simulink model "Model_TranslationEngine64"  (R2022b)
settings: Solver=FixedStepDiscrete  StartTime=0.0  StopTime=5  RelTol=1e-3  EnableMultiTasking=on
InitFcn:
  | % Initialize model
  | ModelSettings=BTConfig.GetModelSettings();
  | 
  | ModelSettings.Validate();
  | 
  | ModelInit;
  | 
  | 
  | % load library data
  | GainLibrary_data;
  | % Load saved values from partition process
  | CapturedConstMask.LoadMapFromFile(bdroot)
StartFcn:
  | % make sure all the simulated RTC requests are found
  | %RTC_SIM_OBJ.ValidateREQs();
undefined symbols (not defined in the file or in its folder): AA, BPLP, Column, NumHFRefBPF, NumHFRefLPF, NumMusicChannels, Row, VolumeMuteConfig
libraries: TuneVar x925, TOP x490, FeaturePath x111, CapturedConstLib x52
(part 25 of 34)

== system Model_TranslationEngine64/ModelPreAmp/DecRate/AudioPilot35/Audiopilot_3_5/NoiseEstimationVariant/RegularNoiseEstimation/LFNoiseEstimatorCoh/SpeedBoundsAndNoiseSlew/LfNoiseSlew ==
  Attack : Subsystem
  Decay : Subsystem
  FeaturePath : FeaturePath/FeaturePath  FeatureName=Slew  IsGroup=off  GroupNumber=-1  IsModule=off  TriggerInit=[-225 44 -110 151]
      settings: SourceProductName=Bose Talaria
  SlowSlew : Subsystem
  Threshold : Subsystem  mask(Talaria Trivial Tune TOP){TriggerInit=[-265 255 -95 285], TopName=ThresholdDb, TuneName=ThresholdDb, DataTypeOut=single, MaskValue=Config.SlewThresholdDb, TunabilityNumber=1, MinValue=[], MaxValue=[], BankNumber=0, PreOverlay=false, PostOverlay=false, UseSameName=on}
      mask prompts: TriggerInit "Hidden: MoveFcn redraw"; TopName "Name:"; TuneName "Name of TuneVar:"; DataTypeOut "Data type:"; MaskValue "Default Value:"; TunabilityNumber "Tunability:"; MinValue "Min Value:"; MaxValue "Max Value:"; BankNumber "Target memory bank number:"; PreOverlay "Requires pre-overlay action:"; PostOverlay "Requires post-overlay action:"; UseSameName "Use same name for tune variable and TOP"
      mask help: The TuneTOP block encapsultes a Target Overlay Parameter, a Tune Variable, and a Trivial Translation between them.
      mask init:
      | [ok,activeTopPath,activeTunePath] = TuneTOP_Mask.Init(gcbh);
      settings: MoveFcn=TuneTOP_Mask.CB_TriggerInit(gcbh);
      mask Callback TriggerInit: TuneTOP_Mask.CB_TriggerInit(gcbh);
      mask TypeOptions TopName: TOP/TopName
      mask TypeOptions TuneName: Tune Variable/TuneName
      mask TypeOptions DataTypeOut: TOP/DataTypeOut
      mask TypeOptions MaskValue: Tune Variable/MaskValue
      mask TypeOptions TunabilityNumber: Tune Variable/TunabilityNumber
      mask Callback TunabilityNumber: TuneVarMask.CB_TunabilityNumber(gcbh);
      mask TypeOptions MinValue: Tune Variable/MinValue
      mask TypeOptions MaxValue: Tune Variable/MaxValue
      mask TypeOptions BankNumber: TOP/BankNumber
      mask TypeOptions PreOverlay: TOP/PreOverlay
      mask TypeOptions PostOverlay: TOP/PostOverlay
      mask Callback UseSameName: TuneTOP_Mask.CB_UseSameName(gcbh);
      mask DialogControl toolPanel Prompt: Tuning Tool Hints
      mask DialogControl DescriptionGroup Prompt: Description
      mask DialogControl EditDescription Prompt: Edit Description
      mask DialogControl EditDescription Callback: TuneTOP_Mask.CB_EditDescription(gcbh);
      mask DialogControl TunabilityText Prompt: Easy: Changes nearly every tuning.
      mask DialogControl AdvancedPanel Prompt: Advanced
      mask DialogControl ConvertToFullTranslation Prompt: Irreversible conversion to full translation
      mask DialogControl ConvertToFullTranslation Callback: TuneTOP_Mask.CB_ConvertToFullTranslation(gcbh);
      mask DialogControl ErrorContainer Prompt: Error Messages
      mask DialogControl ErrorText Prompt: No overlay group found. Declare one in a FeaturePath.
      mask Display:
      | % retrieve icon definition
      | [path,w,h] = TuneTOP_Mask.Icon();
      | 
      | % retrieve the block's pixel size
      | pos = get(gcbh,'position');
      | bw = pos(3) - pos(1);
      | bh = pos(4) - pos(2);
      | 
      | % draw centered icon
      | xAdj = bw/2 - w/2 + 5;
      | yAdj = bh/2 - h/2 + 4;
      | for i=1:length(path)
      | 	patch(path(i).x+xAdj, path(i).y+yAdj, path(i).rgb);
      | end
      | 
      | % show the top name or an X
      | if (exist('ok','var') && ok)
      | 	text(bw*0.5, bh*0.2, activeTopPath, 'horizontalAlignment', 'center');
      | 	patch(0,0,[1 1 1]);
      | 	patch(bw,bh,[1 1 1]);
      | else
      | 	tx=bw*0.03;
      | 	ty=bh*0.03;
      | 	patch([0 tx bw bw-tx], [ty 0 bh-ty bh], [1 0 0]);
      | 	patch([0 bw-tx bw tx], [bh-ty 0 ty bh], [1 0 0]);
      | end

== system Model_TranslationEngine64/ModelPreAmp/DecRate/AudioPilot35/Audiopilot_3_5/NoiseEstimationVariant/RegularNoiseEstimation/LFNoiseEstimatorCoh/SpeedBoundsAndNoiseSlew/SpeedBounds ==
  FeaturePath : FeaturePath/FeaturePath  FeatureName=SpeedBounds  IsGroup=off  GroupNumber=-1  IsModule=off  TriggerInit=[115 194 230 301]
      settings: SourceProductName=Bose Talaria
  axis : Subsystem  mask(Talaria Trivial Tune TOP){TriggerInit=[85 375 255 405], TopName=Axis, TuneName=Axis, DataTypeOut=single, MaskValue=Config.SpeedBoundsAxis, TunabilityNumber=1, MinValue=[], MaxValue=[], BankNumber=0, PreOverlay=false, PostOverlay=false, UseSameName=on}
      mask prompts: TriggerInit "Hidden: MoveFcn redraw"; TopName "Name:"; TuneName "Name of TuneVar:"; DataTypeOut "Data type:"; MaskValue "Default Value:"; TunabilityNumber "Tunability:"; MinValue "Min Value:"; MaxValue "Max Value:"; BankNumber "Target memory bank number:"; PreOverlay "Requires pre-overlay action:"; PostOverlay "Requires post-overlay action:"; UseSameName "Use same name for tune variable and TOP"
      mask help: The TuneTOP block encapsultes a Target Overlay Parameter, a Tune Variable, and a Trivial Translation between them.
      mask init:
      | [ok,activeTopPath,activeTunePath] = TuneTOP_Mask.Init(gcbh);
      settings: MoveFcn=TuneTOP_Mask.CB_TriggerInit(gcbh);
      mask Callback TriggerInit: TuneTOP_Mask.CB_TriggerInit(gcbh);
      mask TypeOptions TopName: TOP/TopName
      mask TypeOptions TuneName: Tune Variable/TuneName
      mask TypeOptions DataTypeOut: TOP/DataTypeOut
      mask TypeOptions MaskValue: Tune Variable/MaskValue
      mask TypeOptions TunabilityNumber: Tune Variable/TunabilityNumber
      mask Callback TunabilityNumber: TuneVarMask.CB_TunabilityNumber(gcbh);
      mask TypeOptions MinValue: Tune Variable/MinValue
      mask TypeOptions MaxValue: Tune Variable/MaxValue
      mask TypeOptions BankNumber: TOP/BankNumber
      mask TypeOptions PreOverlay: TOP/PreOverlay
      mask TypeOptions PostOverlay: TOP/PostOverlay
      mask Callback UseSameName: TuneTOP_Mask.CB_UseSameName(gcbh);
      mask DialogControl toolPanel Prompt: Tuning Tool Hints
      mask DialogControl DescriptionGroup Prompt: Description
      mask DialogControl EditDescription Prompt: Edit Description
      mask DialogControl EditDescription Callback: TuneTOP_Mask.CB_EditDescription(gcbh);
      mask DialogControl TunabilityText Prompt: Easy: Changes nearly every tuning.
      mask DialogControl AdvancedPanel Prompt: Advanced
      mask DialogControl ConvertToFullTranslation Prompt: Irreversible conversion to full translation
      mask DialogControl ConvertToFullTranslation Callback: TuneTOP_Mask.CB_ConvertToFullTranslation(gcbh);
      mask DialogControl ErrorContainer Prompt: Error Messages
      mask DialogControl ErrorText Prompt: No overlay group found. Declare one in a FeaturePath.
      mask Display:
      | % retrieve icon definition
      | [path,w,h] = TuneTOP_Mask.Icon();
      | 
      | % retrieve the block's pixel size
      | pos = get(gcbh,'position');
      | bw = pos(3) - pos(1);
      | bh = pos(4) - pos(2);
      | 
      | % draw centered icon
      | xAdj = bw/2 - w/2 + 5;
      | yAdj = bh/2 - h/2 + 4;
      | for i=1:length(path)
      | 	patch(path(i).x+xAdj, path(i).y+yAdj, path(i).rgb);
      | end
      | 
      | % show the top name or an X
      | if (exist('ok','var') && ok)
      | 	text(bw*0.5, bh*0.2, activeTopPath, 'horizontalAlignment', 'center');
      | 	patch(0,0,[1 1 1]);
      | 	patch(bw,bh,[1 1 1]);
      | else
      | 	tx=bw*0.03;
      | 	ty=bh*0.03;
      | 	patch([0 tx bw bw-tx], [ty 0 bh-ty bh], [1 0 0]);
      | 	patch([0 bw-tx bw tx], [bh-ty 0 ty bh], [1 0 0]);
      | end
  max : Subsystem  mask(Talaria Trivial Tune TOP){TriggerInit=[85 485 255 515], TopName=MaxDbspl, TuneName=MaxDbspl, DataTypeOut=single, MaskValue=Config.SpeedBoundsMaxdBSPL, TunabilityNumber=1, MinValue=[], MaxValue=[], BankNumber=0, PreOverlay=false, PostOverlay=false, UseSameName=on}
      mask prompts: TriggerInit "Hidden: MoveFcn redraw"; TopName "Name:"; TuneName "Name of TuneVar:"; DataTypeOut "Data type:"; MaskValue "Default Value:"; TunabilityNumber "Tunability:"; MinValue "Min Value:"; MaxValue "Max Value:"; BankNumber "Target memory bank number:"; PreOverlay "Requires pre-overlay action:"; PostOverlay "Requires post-overlay action:"; UseSameName "Use same name for tune variable and TOP"
      mask help: The TuneTOP block encapsultes a Target Overlay Parameter, a Tune Variable, and a Trivial Translation between them.
      mask init:
      | [ok,activeTopPath,activeTunePath] = TuneTOP_Mask.Init(gcbh);
      settings: MoveFcn=TuneTOP_Mask.CB_TriggerInit(gcbh);
      mask Callback TriggerInit: TuneTOP_Mask.CB_TriggerInit(gcbh);
      mask TypeOptions TopName: TOP/TopName
      mask TypeOptions TuneName: Tune Variable/TuneName
      mask TypeOptions DataTypeOut: TOP/DataTypeOut
      mask TypeOptions MaskValue: Tune Variable/MaskValue
      mask TypeOptions TunabilityNumber: Tune Variable/TunabilityNumber
      mask Callback TunabilityNumber: TuneVarMask.CB_TunabilityNumber(gcbh);
      mask TypeOptions MinValue: Tune Variable/MinValue
      mask TypeOptions MaxValue: Tune Variable/MaxValue
      mask TypeOptions BankNumber: TOP/BankNumber
      mask TypeOptions PreOverlay: TOP/PreOverlay
      mask TypeOptions PostOverlay: TOP/PostOverlay
      mask Callback UseSameName: TuneTOP_Mask.CB_UseSameName(gcbh);
      mask DialogControl toolPanel Prompt: Tuning Tool Hints
      mask DialogControl DescriptionGroup Prompt: Description
      mask DialogControl EditDescription Prompt: Edit Description
      mask DialogControl EditDescription Callback: TuneTOP_Mask.CB_EditDescription(gcbh);
      mask DialogControl TunabilityText Prompt: Easy: Changes nearly every tuning.
      mask DialogControl AdvancedPanel Prompt: Advanced
      mask DialogControl ConvertToFullTranslation Prompt: Irreversible conversion to full translation
      mask DialogControl ConvertToFullTranslation Callback: TuneTOP_Mask.CB_ConvertToFullTranslation(gcbh);
      mask DialogControl ErrorContainer Prompt: Error Messages
      mask DialogControl ErrorText Prompt: No overlay group found. Declare one in a FeaturePath.
      mask Display:
      | % retrieve icon definition
      | [path,w,h] = TuneTOP_Mask.Icon();
      | 
      | % retrieve the block's pixel size
      | pos = get(gcbh,'position');
      | bw = pos(3) - pos(1);
      | bh = pos(4) - pos(2);
      | 
      | % draw centered icon
      | xAdj = bw/2 - w/2 + 5;
      | yAdj = bh/2 - h/2 + 4;
      | for i=1:length(path)
      | 	patch(path(i).x+xAdj, path(i).y+yAdj, path(i).rgb);
      | end
      | 
      | % show the top name or an X
      | if (exist('ok','var') && ok)
      | 	text(bw*0.5, bh*0.2, activeTopPath, 'horizontalAlignment', 'center');
      | 	patch(0,0,[1 1 1]);
      | 	patch(bw,bh,[1 1 1]);
      | else
      | 	tx=bw*0.03;
      | 	ty=bh*0.03;
      | 	patch([0 tx bw bw-tx], [ty 0 bh-ty bh], [1 0 0]);
      | 	patch([0 bw-tx bw tx], [bh-ty 0 ty bh], [1 0 0]);
      | end
  min : Subsystem
  on : Subsystem  mask(Talaria Trivial Tune TOP){TriggerInit=[85 540 255 570], TopName=On, TuneName=On, DataTypeOut=single, MaskValue=Config.SpeedBoundsOn, TunabilityNumber=1, MinValue=[], MaxValue=[], BankNumber=0, PreOverlay=false, PostOverlay=false, UseSameName=on}
      mask prompts: TriggerInit "Hidden: MoveFcn redraw"; TopName "Name:"; TuneName "Name of TuneVar:"; DataTypeOut "Data type:"; MaskValue "Default Value:"; TunabilityNumber "Tunability:"; MinValue "Min Value:"; MaxValue "Max Value:"; BankNumber "Target memory bank number:"; PreOverlay "Requires pre-overlay action:"; PostOverlay "Requires post-overlay action:"; UseSameName "Use same name for tune variable and TOP"
      mask help: The TuneTOP block encapsultes a Target Overlay Parameter, a Tune Variable, and a Trivial Translation between them.
      mask init:
      | [ok,activeTopPath,activeTunePath] = TuneTOP_Mask.Init(gcbh);
      settings: MoveFcn=TuneTOP_Mask.CB_TriggerInit(gcbh);
      mask Callback TriggerInit: TuneTOP_Mask.CB_TriggerInit(gcbh);
      mask TypeOptions TopName: TOP/TopName
      mask TypeOptions TuneName: Tune Variable/TuneName
      mask TypeOptions DataTypeOut: TOP/DataTypeOut
      mask TypeOptions MaskValue: Tune Variable/MaskValue
      mask TypeOptions TunabilityNumber: Tune Variable/TunabilityNumber
      mask Callback TunabilityNumber: TuneVarMask.CB_TunabilityNumber(gcbh);
      mask TypeOptions MinValue: Tune Variable/MinValue
      mask TypeOptions MaxValue: Tune Variable/MaxValue
      mask TypeOptions BankNumber: TOP/BankNumber
      mask TypeOptions PreOverlay: TOP/PreOverlay
      mask TypeOptions PostOverlay: TOP/PostOverlay
      mask Callback UseSameName: TuneTOP_Mask.CB_UseSameName(gcbh);
      mask DialogControl toolPanel Prompt: Tuning Tool Hints
      mask DialogControl DescriptionGroup Prompt: Description
      mask DialogControl EditDescription Prompt: Edit Description
      mask DialogControl EditDescription Callback: TuneTOP_Mask.CB_EditDescription(gcbh);
      mask DialogControl TunabilityText Prompt: Easy: Changes nearly every tuning.
      mask DialogControl AdvancedPanel Prompt: Advanced
      mask DialogControl ConvertToFullTranslation Prompt: Irreversible conversion to full translation
      mask DialogControl ConvertToFullTranslation Callback: TuneTOP_Mask.CB_ConvertToFullTranslation(gcbh);
      mask DialogControl ErrorContainer Prompt: Error Messages
      mask DialogControl ErrorText Prompt: No overlay group found. Declare one in a FeaturePath.
      mask Display:
      | % retrieve icon definition
      | [path,w,h] = TuneTOP_Mask.Icon();
      | 
      | % retrieve the block's pixel size
      | pos = get(gcbh,'position');
      | bw = pos(3) - pos(1);
      | bh = pos(4) - pos(2);
      | 
      | % draw centered icon
      | xAdj = bw/2 - w/2 + 5;
      | yAdj = bh/2 - h/2 + 4;
      | for i=1:length(path)
      | 	patch(path(i).x+xAdj, path(i).y+yAdj, path(i).rgb);
      | end
      | 
      | % show the top name or an X
      | if (exist('ok','var') && ok)
      | 	text(bw*0.5, bh*0.2, activeTopPath, 'horizontalAlignment', 'center');
      | 	patch(0,0,[1 1 1]);
      | 	patch(bw,bh,[1 1 1]);
      | else
      | 	tx=bw*0.03;
      | 	ty=bh*0.03;
      | 	patch([0 tx bw bw-tx], [ty 0 bh-ty bh], [1 0 0]);
      | 	patch([0 bw-tx bw tx], [bh-ty 0 ty bh], [1 0 0]);
      | end

== system Model_TranslationEngine64/ModelPreAmp/DecRate/AudioPilot35/Audiopilot_3_5/NoiseEstimationVariant/RegularNoiseEstimation/RatioCalculation/APLFUP/FlagHoldTime ==
  TOP : TOP/TOP  TriggerInit=[435 27 630 73]  TopName=FlagHoldTimeSamples  DataTypeOut=single  BankNumber=0  PreOverlay=false  PostOverlay=false  Role=Automatic
      settings: SourceProductName=Bose Talaria
  TranslateTrigger : TuneVar/TranslateTrigger  TriggerInit=[306 -100 344 -45]
      settings: SourceProductName=Bose Talaria
  Tune Variable : TuneVar/TuneVar  TuneName=FlagHoldTimeS  SpecifyMaxSize=off  VariableDim=1 (Row)  MaxSize=[1 1]  TunabilityNumber=1  MinValue=[]  MaxValue=[]  TriggerInit=[-35 27 160 73]  MaskValue=Config.UpdateFlagHoldTimeSec
      settings: SourceProductName=Bose Talaria
  sec2samples : MATLAB Function  TreatAsAtomicUnit=on
  wires:
  Tune Variable/1 -> sec2samples/1(time)  "FlagHoldTimeS"
  sec2samples/1(samples) -> TOP/1
  TranslateTrigger/1 -> sec2samples/Trigger

== system Model_TranslationEngine64/ModelPreAmp/DecRate/AudioPilot35/Audiopilot_3_5/NoiseEstimationVariant/RegularNoiseEstimation/RatioCalculation/APLFUP/HfNoiseThresh ==
  TOP : TOP/TOP  TriggerInit=[440 20 585 80]  TopName=HfNoiseThreshDbspl  DataTypeOut=single  BankNumber=BankNumber  PreOverlay=PreOverlay  PostOverlay=PostOverlay  Role=Automatic
      settings: SourceProductName=Bose Talaria
  TrivialTranslation : TuneVar/TrivialTranslation  TriggerInit=[300 28 350 72]
      settings: SourceProductName=Bose Talaria
  Tune Variable : TuneVar/TuneVar  TuneName=HfNoiseThreshDbspl  SpecifyMaxSize=off  VariableDim=1 (Row)  MaxSize=[1 1]  TunabilityNumber=1  MinValue=MinValue  MaxValue=MaxValue  TriggerInit=[20 25 190 75]  MaskValue=MaskValue
      settings: SourceProductName=Bose Talaria
  wires:
  TrivialTranslation/1 -> TOP/1
  Tune Variable/1 -> TrivialTranslation/1  "HfNoiseThreshDbspl"

== system Model_TranslationEngine64/ModelPreAmp/DecRate/AudioPilot35/Audiopilot_3_5/NoiseEstimationVariant/RegularNoiseEstimation/RatioCalculation/APLFUP/LfNoiseThresh ==
  TOP : TOP/TOP  TriggerInit=[440 20 585 80]  TopName=LfNoiseThreshDbspl  DataTypeOut=single  BankNumber=BankNumber  PreOverlay=PreOverlay  PostOverlay=PostOverlay  Role=Automatic
      settings: SourceProductName=Bose Talaria
  TrivialTranslation : TuneVar/TrivialTranslation  TriggerInit=[300 28 350 72]
      settings: SourceProductName=Bose Talaria
  Tune Variable : TuneVar/TuneVar  TuneName=LfNoiseThreshDbspl  SpecifyMaxSize=off  VariableDim=1 (Row)  MaxSize=[1 1]  TunabilityNumber=1  MinValue=MinValue  MaxValue=MaxValue  TriggerInit=[20 25 190 75]  MaskValue=MaskValue
      settings: SourceProductName=Bose Talaria
  wires:
  TrivialTranslation/1 -> TOP/1
  Tune Variable/1 -> TrivialTranslation/1  "LfNoiseThreshDbspl"

== system Model_TranslationEngine64/ModelPreAmp/DecRate/AudioPilot35/Audiopilot_3_5/NoiseEstimationVariant/RegularNoiseEstimation/RatioCalculation/APLFUP/LfNoiseUpdatePeriod ==
  TOP : TOP/TOP  TriggerInit=[440 20 685 80]  TopName=LfNoiseUpdatePeriodSamples  DataTypeOut=single  BankNumber=0  PreOverlay=false  PostOverlay=false  Role=Automatic
      settings: SourceProductName=Bose Talaria
  TranslateTrigger : TuneVar/TranslateTrigger  TriggerInit=[306 -100 344 -45]
      settings: SourceProductName=Bose Talaria
  Tune Variable : TuneVar/TuneVar  TuneName=LfNoiseUpdatePeriodS  SpecifyMaxSize=off  VariableDim=1 (Row)  MaxSize=[1 1]  TunabilityNumber=1  MinValue=[]  MaxValue=[]  TriggerInit=[-100 20 145 80]  MaskValue=Config.UpdateLfNoiseUpdatePeriodSec
      settings: SourceProductName=Bose Talaria
  sec2samples : MATLAB Function  TreatAsAtomicUnit=on
  wires:
  Tune Variable/1 -> sec2samples/1(time)  "LfNoiseUpdatePeriodS"
  sec2samples/1(samples) -> TOP/1
  TranslateTrigger/1 -> sec2samples/Trigger

== system Model_TranslationEngine64/ModelPreAmp/DecRate/AudioPilot35/Audiopilot_3_5/NoiseEstimationVariant/RegularNoiseEstimation/RatioCalculation/APLFUP/LfNoiseUpdateThresh ==
  TOP : TOP/TOP  TriggerInit=[440 20 585 80]  TopName=LfNoiseUpdateThreshDb  DataTypeOut=single  BankNumber=BankNumber  PreOverlay=PreOverlay  PostOverlay=PostOverlay  Role=Automatic
      settings: SourceProductName=Bose Talaria
  TrivialTranslation : TuneVar/TrivialTranslation  TriggerInit=[300 28 350 72]
      settings: SourceProductName=Bose Talaria
  Tune Variable : TuneVar/TuneVar  TuneName=LfNoiseUpdateThreshDb  SpecifyMaxSize=off  VariableDim=1 (Row)  MaxSize=[1 1]  TunabilityNumber=1  MinValue=MinValue  MaxValue=MaxValue  TriggerInit=[20 25 190 75]  MaskValue=MaskValue
      settings: SourceProductName=Bose Talaria
  wires:
  TrivialTranslation/1 -> TOP/1
  Tune Variable/1 -> TrivialTranslation/1  "LfNoiseUpdateThreshDb"

== system Model_TranslationEngine64/ModelPreAmp/DecRate/AudioPilot35/Audiopilot_3_5/NoiseEstimationVariant/RegularNoiseEstimation/RatioCalculation/APLFUP/SpeedUpdateThresh ==
  TOP : TOP/TOP  TriggerInit=[440 20 585 80]  TopName=SpeedUpdateThreshMph  DataTypeOut=single  BankNumber=BankNumber  PreOverlay=PreOverlay  PostOverlay=PostOverlay  Role=Automatic
      settings: SourceProductName=Bose Talaria
  TrivialTranslation : TuneVar/TrivialTranslation  TriggerInit=[300 28 350 72]
      settings: SourceProductName=Bose Talaria
  Tune Variable : TuneVar/TuneVar  TuneName=SpeedUpdateThreshMph  SpecifyMaxSize=off  VariableDim=1 (Row)  MaxSize=[1 1]  TunabilityNumber=1  MinValue=MinValue  MaxValue=MaxValue  TriggerInit=[20 25 190 75]  MaskValue=MaskValue
      settings: SourceProductName=Bose Talaria
  wires:
  TrivialTranslation/1 -> TOP/1
  Tune Variable/1 -> TrivialTranslation/1  "SpeedUpdateThreshMph"

== system Model_TranslationEngine64/ModelPreAmp/DecRate/AudioPilot35/Audiopilot_3_5/NoiseEstimationVariant/RegularNoiseEstimation/RatioCalculation/RatioSlew/attack ==
  TOP : TOP/TOP  TriggerInit=[-10 87 195 133]  TopName=AttackDbPerSample  DataTypeOut=single  BankNumber=0  PreOverlay=false  PostOverlay=false  Role=Automatic
      settings: SourceProductName=Bose Talaria
  TranslateTrigger : TuneVar/TranslateTrigger  TriggerInit=[-119 -30 -81 25]
      settings: SourceProductName=Bose Talaria
  Tune Variable : TuneVar/TuneVar  TuneName=AttackDbPerS  SpecifyMaxSize=off  VariableDim=1 (Row)  MaxSize=[1 1]  TunabilityNumber=1  MinValue=[]  MaxValue=[]  TriggerInit=[-475 85 -305 135]  MaskValue=Config.SlewAttackDbpersec
      settings: SourceProductName=Bose Talaria
  sec2sample : MATLAB Function  TreatAsAtomicUnit=on
  wires:
  sec2sample/1(y) -> TOP/1
  Tune Variable/1 -> sec2sample/1(u)  "AttackDbPerS"
  TranslateTrigger/1 -> sec2sample/Trigger

== system Model_TranslationEngine64/ModelPreAmp/DecRate/AudioPilot35/Audiopilot_3_5/NoiseEstimationVariant/RegularNoiseEstimation/RatioCalculation/RatioSlew/decay ==
  TOP : TOP/TOP  TriggerInit=[-15 85 195 135]  TopName=DecayDbPerSample  DataTypeOut=single  BankNumber=0  PreOverlay=false  PostOverlay=false  Role=Automatic
      settings: SourceProductName=Bose Talaria
  TranslateTrigger : TuneVar/TranslateTrigger  TriggerInit=[-119 -30 -81 25]
      settings: SourceProductName=Bose Talaria
  Tune Variable : TuneVar/TuneVar  TuneName=DecayDbPerS  SpecifyMaxSize=off  VariableDim=1 (Row)  MaxSize=[1 1]  TunabilityNumber=1  MinValue=[]  MaxValue=[]  TriggerInit=[-485 85 -315 135]  MaskValue=Config.SlewDecayDbpersec
      settings: SourceProductName=Bose Talaria
  sec2sample : MATLAB Function  TreatAsAtomicUnit=on
  wires:
  TranslateTrigger/1 -> sec2sample/Trigger
  Tune Variable/1 -> sec2sample/1(u)  "DecayDbPerS"
  sec2sample/1(y) -> TOP/1

== system Model_TranslationEngine64/ModelPreAmp/DecRate/AudioPilot35/Audiopilot_3_5/NoiseEstimationVariant/RegularNoiseEstimation/RatioCalculation/RatioSlew/threshold ==
  TOP : TOP/TOP  TriggerInit=[440 20 585 80]  TopName=ThresholdDb  DataTypeOut=single  BankNumber=BankNumber  PreOverlay=PreOverlay  PostOverlay=PostOverlay  Role=Automatic
      settings: SourceProductName=Bose Talaria
  TrivialTranslation : TuneVar/TrivialTranslation  TriggerInit=[300 28 350 72]
      settings: SourceProductName=Bose Talaria
  Tune Variable : TuneVar/TuneVar  TuneName=ThresholdDb  SpecifyMaxSize=off  VariableDim=1 (Row)  MaxSize=[1 1]  TunabilityNumber=1  MinValue=MinValue  MaxValue=MaxValue  TriggerInit=[20 25 190 75]  MaskValue=MaskValue
      settings: SourceProductName=Bose Talaria
  wires:
  TrivialTranslation/1 -> TOP/1
  Tune Variable/1 -> TrivialTranslation/1  "ThresholdDb"

== system Model_TranslationEngine64/ModelPreAmp/DecRate/AudioPilot35/Audiopilot_3_5/NoiseEstimationVariant/RegularNoiseEstimation/RatioCalculation/RatioSmoother/RatioImpulseRejectionGamma0 ==
  TOP : TOP/TOP  TriggerInit=[440 20 725 80]  TopName=Gamma0  DataTypeOut=single  BankNumber=0  PreOverlay=false  PostOverlay=false  Role=Automatic
      settings: SourceProductName=Bose Talaria
  Tau2Gamma : MATLAB Function  TreatAsAtomicUnit=on
  TranslateTrigger : TuneVar/TranslateTrigger  TriggerInit=[306 -100 344 -45]
      settings: SourceProductName=Bose Talaria
  Tune Variable : TuneVar/TuneVar  TuneName=Gamma0TauS  SpecifyMaxSize=off  VariableDim=1 (Row)  MaxSize=[1 1]  TunabilityNumber=1  MinValue=[]  MaxValue=[]  TriggerInit=[-195 25 60 75]  MaskValue=Config.ImpRejGamma0TauSec
      settings: SourceProductName=Bose Talaria
  wires:
  Tune Variable/1 -> Tau2Gamma/1(tau)  "Gamma0TauS"
  Tau2Gamma/1(gamma) -> TOP/1
  TranslateTrigger/1 -> Tau2Gamma/Trigger

== system Model_TranslationEngine64/ModelPreAmp/DecRate/AudioPilot35/Audiopilot_3_5/NoiseEstimationVariant/RegularNoiseEstimation/RatioCalculation/RatioSmoother/RatioImpulseRejectionImpulseVarianceLpfCoef ==
  TOP : TOP/TOP  TriggerInit=[285 19 540 81]  TopName=ImpulseVarianceLpfCoef  DataTypeOut=single  BankNumber=0  PreOverlay=false  PostOverlay=false  Role=Automatic
      settings: SourceProductName=Bose Talaria
  Tau2Coef : MATLAB Function  TreatAsAtomicUnit=on
  TranslateTrigger : TuneVar/TranslateTrigger  TriggerInit=[151 -115 189 -60]
      settings: SourceProductName=Bose Talaria
  Tune Variable : TuneVar/TuneVar  TuneName=ImpulseVarianceLpfTauS  SpecifyMaxSize=off  VariableDim=1 (Row)  MaxSize=[1 1]  TunabilityNumber=1  MinValue=[]  MaxValue=[]  TriggerInit=[-275 19 -20 81]  MaskValue=Config.ImpRejImpulseVarianceLpfTauSec
      settings: SourceProductName=Bose Talaria
  wires:
  Tune Variable/1 -> Tau2Coef/1(tau)  "ImpulseVarianceLpfTauS"
  Tau2Coef/1(coef) -> TOP/1
  TranslateTrigger/1 -> Tau2Coef/Trigger

== system Model_TranslationEngine64/ModelPreAmp/DecRate/AudioPilot35/Audiopilot_3_5/NoiseEstimationVariant/RegularNoiseEstimation/RatioCalculation/RatioSmoother/RatioImpulseRejectionImpulseVarianceScale ==
  TOP : TOP/TOP  TriggerInit=[440 20 585 80]  TopName=ImpulseVarianceScale  DataTypeOut=single  BankNumber=BankNumber  PreOverlay=PreOverlay  PostOverlay=PostOverlay  Role=Automatic
      settings: SourceProductName=Bose Talaria
  TrivialTranslation : TuneVar/TrivialTranslation  TriggerInit=[300 28 350 72]
      settings: SourceProductName=Bose Talaria
  Tune Variable : TuneVar/TuneVar  TuneName=ImpulseVarianceScale  SpecifyMaxSize=off  VariableDim=1 (Row)  MaxSize=[1 1]  TunabilityNumber=1  MinValue=MinValue  MaxValue=MaxValue  TriggerInit=[20 25 190 75]  MaskValue=MaskValue
      settings: SourceProductName=Bose Talaria
  wires:
  TrivialTranslation/1 -> TOP/1
  Tune Variable/1 -> TrivialTranslation/1  "ImpulseVarianceScale"

== system Model_TranslationEngine64/ModelPreAmp/DecRate/AudioPilot35/Audiopilot_3_5/NoiseEstimationVariant/RegularNoiseEstimation/RatioCalculation/RatioSmoother/RatioImpulseRejectionNoiseVarianceScale ==
  TOP : TOP/TOP  TriggerInit=[440 20 585 80]  TopName=NoiseVarianceScale  DataTypeOut=single  BankNumber=BankNumber  PreOverlay=PreOverlay  PostOverlay=PostOverlay  Role=Automatic
      settings: SourceProductName=Bose Talaria
  TrivialTranslation : TuneVar/TrivialTranslation  TriggerInit=[300 28 350 72]
      settings: SourceProductName=Bose Talaria
  Tune Variable : TuneVar/TuneVar  TuneName=NoiseVarianceScale  SpecifyMaxSize=off  VariableDim=1 (Row)  MaxSize=[1 1]  TunabilityNumber=1  MinValue=MinValue  MaxValue=MaxValue  TriggerInit=[20 25 190 75]  MaskValue=MaskValue
      settings: SourceProductName=Bose Talaria
  wires:
  TrivialTranslation/1 -> TOP/1
  Tune Variable/1 -> TrivialTranslation/1  "NoiseVarianceScale"

== system Model_TranslationEngine64/ModelPreAmp/DecRate/Medusa5H1/MedusaHoligram/Medusa5H1 Part 2/Decimated-Rate FDP/Fdp/FreqDomainProcessing/CalculateAndApplyCoefficients ==
  note: 1) Add Subsystem or Model blocks as valid variant choices.
      | 2) You cannot connect blocks at this level. At simulation, connectivity is automatically
      | determined, based on the active variant and port name matching.
  DeciRate : Subsystem  VariantControl="Config.Variant == \"DeciRate\""
  FullRate : Subsystem  VariantControl="Config.Variant == \"FullRate\""

== system Model_TranslationEngine64/ModelPreAmp/DecRate/Medusa5H1/MedusaHoligram/Medusa5H1 Part 2/Decimated-Rate FDP/Fdp/FreqDomainProcessing/Reverb Extractions ==
  note: Rate Transition blocks are inserted after TOPs to convert their sample rate
      | to decimated rate. Initially their sample rate is inherited from the fastest one
      | of all the blocks that use it, which happen to be inside full-rate processing.
  Captured Tune Const : CapturedConstLib/CapturedConst  TriggerInit=[200 -98 300 -62]  Role=Automatic
      settings: SourceProductName=Bose Talaria
  Captured Tune Const1 : CapturedConstLib/CapturedConst  TriggerInit=[200 -38 300 -2]  Role=Automatic
      settings: SourceProductName=Bose Talaria
  FeaturePath : FeaturePath/FeaturePath  FeatureName=Spum  IsGroup=off  GroupNumber=-1  IsModule=off  TriggerInit=[-175 -281 -10 -169]
      settings: SourceProductName=Bose Talaria
  TOP : TOP/TOP  TriggerInit=[575 -440 850 -380]  TopName=FastPsdSmoothFactor  DataTypeOut=single  BankNumber=0  PreOverlay=false  PostOverlay=false  Role=Automatic
      settings: SourceProductName=Bose Talaria
  TOP1 : TOP/TOP  TriggerInit=[575 -350 850 -290]  TopName=SlowPsdSmoothFactor  DataTypeOut=single  BankNumber=0  PreOverlay=false  PostOverlay=false  Role=Automatic
      settings: SourceProductName=Bose Talaria
  TOP3 : TOP/TOP  TriggerInit=[575 -110 850 -50]  TopName=DirectPathSamplesDec  DataTypeOut=single  BankNumber=0  PreOverlay=false  PostOverlay=false  Role=Automatic
      settings: SourceProductName=Bose Talaria
  TOP4 : TOP/TOP  TriggerInit=[580 -658 845 -592]  TopName=LsSmoothFactor  DataTypeOut=single  BankNumber=0  PreOverlay=false  PostOverlay=false  Role=Automatic
      settings: SourceProductName=Bose Talaria
  TranslateTrigger1 : TuneVar/TranslateTrigger  TriggerInit=[421 -535 459 -480]
      settings: SourceProductName=Bose Talaria
  TranslateTrigger3 : TuneVar/TranslateTrigger  TriggerInit=[421 -245 459 -190]
      settings: SourceProductName=Bose Talaria
  TranslateTrigger4 : TuneVar/TranslateTrigger  TriggerInit=[421 -765 459 -710]
      settings: SourceProductName=Bose Talaria
  Trivial Translation1 : MATLAB Function  TreatAsAtomicUnit=on
  Trivial Translation3 : MATLAB Function  TreatAsAtomicUnit=on
  Trivial Translation4 : MATLAB Function  TreatAsAtomicUnit=on
  wires:
  TranslateTrigger3/1 -> Trivial Translation3/Trigger
  Trivial Translation3/1(DirectPathDec) -> TOP3/1
  [DirectPathSec] -> Trivial Translation3/1(DirectPathSec)
  [SlowPsdSmoothCutoff] -> Trivial Translation1/2(SlowPsdSmoothCutoff)  "variable"
  TranslateTrigger1/1 -> Trivial Translation1/Trigger
  Trivial Translation1/2(SlowPsdSmoothFactor) -> TOP1/1
  [LsSmooth] -> Trivial Translation4/1(LsSmoothCutoff)
  TranslateTrigger4/1 -> Trivial Translation4/Trigger
  Trivial Translation4/1(LsSmoothFactor) -> TOP4/1
  [FastPsdSmoothCutoff] -> Trivial Translation1/1(FastPsdSmoothCutoff)  "variable"
  Trivial Translation1/1(FastPsdSmoothFactor) -> TOP/1
  Captured Tune Const/1 -> Trivial Translation3/2(FrameRate), Trivial Translation4/2(FrameRate), Trivial Translation1/3(FrameRate)
  Captured Tune Const1/1 -> Trivial Translation3/3(FrameSize)

== system Model_TranslationEngine64/ModelPreAmp/DecRate/Medusa5H1/MedusaHoligram/Medusa5H1 Part 2/Full-Rate FDP/Fdp/FreqDomainProcessing/CalculateAndApplyCoefficients ==
  note: 1) Add Subsystem or Model blocks as valid variant choices.
      | 2) You cannot connect blocks at this level. At simulation, connectivity is automatically
      | determined, based on the active variant and port name matching.
  DeciRate : Subsystem  VariantControl="Config.Variant == \"DeciRate\""
  FullRate : Subsystem  VariantControl="Config.Variant == \"FullRate\""

== system Model_TranslationEngine64/ModelPreAmp/DecRate/Medusa5H1/MedusaHoligram/Medusa5H1 Part 2/Full-Rate FDP/Fdp/FreqDomainProcessing/Reverb Extractions ==
  note: Rate Transition blocks are inserted after TOPs to convert their sample rate
      | to decimated rate. Initially their sample rate is inherited from the fastest one
      | of all the blocks that use it, which happen to be inside full-rate processing.
  Captured Tune Const : CapturedConstLib/CapturedConst  TriggerInit=[200 -98 300 -62]  Role=Automatic
      settings: SourceProductName=Bose Talaria
  Captured Tune Const1 : CapturedConstLib/CapturedConst  TriggerInit=[200 -38 300 -2]  Role=Automatic
      settings: SourceProductName=Bose Talaria
  FeaturePath : FeaturePath/FeaturePath  FeatureName=Spum  IsGroup=off  GroupNumber=-1  IsModule=off  TriggerInit=[-175 -281 -10 -169]
      settings: SourceProductName=Bose Talaria
  TOP : TOP/TOP  TriggerInit=[575 -440 850 -380]  TopName=FastPsdSmoothFactor  DataTypeOut=single  BankNumber=0  PreOverlay=false  PostOverlay=false  Role=Automatic
      settings: SourceProductName=Bose Talaria
  TOP1 : TOP/TOP  TriggerInit=[575 -350 850 -290]  TopName=SlowPsdSmoothFactor  DataTypeOut=single  BankNumber=0  PreOverlay=false  PostOverlay=false  Role=Automatic
      settings: SourceProductName=Bose Talaria
  TOP3 : TOP/TOP  TriggerInit=[575 -110 850 -50]  TopName=DirectPathSamplesDec  DataTypeOut=single  BankNumber=0  PreOverlay=false  PostOverlay=false  Role=Automatic
      settings: SourceProductName=Bose Talaria
  TOP4 : TOP/TOP  TriggerInit=[580 -658 845 -592]  TopName=LsSmoothFactor  DataTypeOut=single  BankNumber=0  PreOverlay=false  PostOverlay=false  Role=Automatic
      settings: SourceProductName=Bose Talaria
  TranslateTrigger1 : TuneVar/TranslateTrigger  TriggerInit=[421 -535 459 -480]
      settings: SourceProductName=Bose Talaria
  TranslateTrigger3 : TuneVar/TranslateTrigger  TriggerInit=[421 -245 459 -190]
      settings: SourceProductName=Bose Talaria
  TranslateTrigger4 : TuneVar/TranslateTrigger  TriggerInit=[421 -765 459 -710]
      settings: SourceProductName=Bose Talaria
  Trivial Translation1 : MATLAB Function  TreatAsAtomicUnit=on
  Trivial Translation3 : MATLAB Function  TreatAsAtomicUnit=on
  Trivial Translation4 : MATLAB Function  TreatAsAtomicUnit=on
  wires:
  TranslateTrigger3/1 -> Trivial Translation3/Trigger
  Trivial Translation3/1(DirectPathDec) -> TOP3/1
  [DirectPathSec] -> Trivial Translation3/1(DirectPathSec)
  [SlowPsdSmoothCutoff] -> Trivial Translation1/2(SlowPsdSmoothCutoff)  "variable"
  TranslateTrigger1/1 -> Trivial Translation1/Trigger
  Trivial Translation1/2(SlowPsdSmoothFactor) -> TOP1/1
  [LsSmooth] -> Trivial Translation4/1(LsSmoothCutoff)
  TranslateTrigger4/1 -> Trivial Translation4/Trigger
  Trivial Translation4/1(LsSmoothFactor) -> TOP4/1
  [FastPsdSmoothCutoff] -> Trivial Translation1/1(FastPsdSmoothCutoff)  "variable"
  Trivial Translation1/1(FastPsdSmoothFactor) -> TOP/1
  Captured Tune Const/1 -> Trivial Translation3/2(FrameRate), Trivial Translation4/2(FrameRate), Trivial Translation1/3(FrameRate)
  Captured Tune Const1/1 -> Trivial Translation3/3(FrameSize)

== system Model_TranslationEngine64/ModelPreAmp/DecRate/Medusa5H1/MedusaHoligram/Medusa5H1 Part 2/SPUM Decay Estimate/High-pass filter > 6kHz/InnerLink/PoolIirTunableWithReset ==
  CapturedTuneConst : CapturedConstLib/CapturedConst  TriggerInit=[-600 302 -500 338]  Role=Automatic
      settings: SourceProductName=Bose Talaria
  FeaturePath : FeaturePath/FeaturePath  FeatureName=HPF  IsGroup=off  GroupNumber=-1  IsModule=off  TriggerInit=[-750 -81 -635 26]
      settings: SourceProductName=Bose Talaria
  TOP : TOP/TOP  TriggerInit=[-145 187 5 243]  TopName=PooliirNumStages  DataTypeOut=uint32  BankNumber=0  PreOverlay=false  PostOverlay=Config.VariantObj.PostOverlayRequired  Role=Automatic
      settings: SourceProductName=Bose Talaria
  TOP1 : TOP/TOP  TriggerInit=[-140 277 10 333]  TopName=pooliirCoeffs  DataTypeOut=single  BankNumber=0  PreOverlay=false  PostOverlay=Config.VariantObj.PostOverlayRequired  Role=Automatic
      settings: SourceProductName=Bose Talaria
  TranslateTrigger : TuneVar/TranslateTrigger  TriggerInit=[-339 35 -301 90]
      settings: SourceProductName=Bose Talaria
  Translation : MATLAB Function  TreatAsAtomicUnit=on  mask{MaxNumStages=Config.MaxNumStages, VariantUint8=Config.Variant.Uint8Str}
      mask prompts: VariantUint8 "Variant"
  Tune Variable1 : TuneVar/TuneVar  TuneName=numStages  SpecifyMaxSize=off  VariableDim=1 (Row)  MaxSize=[1 1]  TunabilityNumber=1  MinValue=[]  MaxValue=[]  TriggerInit=[-750 235 -580 285]  MaskValue=Config.TuneDefaults.NumStages
      settings: SourceProductName=Bose Talaria
  Tune Variable2 : TuneVar/TuneVar  TuneName=sosCoefficients  SpecifyMaxSize=on  VariableDim=1 (Row)  MaxSize=[Config.MaxNumStages 6]  TunabilityNumber=1  MinValue=[]  MaxValue=[]  TriggerInit=[-750 175 -580 225]  MaskValue=Config.TuneDefaults.SosCoefficients
      settings: SourceProductName=Bose Talaria
  wires:
  CapturedTuneConst/1 -> Translation/3(NumChannels)
  Tune Variable1/1 -> Translation/2(NumStages)  "numStages"
  Translation/1(PoolNumStages) -> TOP/1
  Translation/2(PoolCoeffs) -> TOP1/1
  Tune Variable2/1 -> Translation/1(RawSOS)  "sosCoefficients"
  TranslateTrigger/1 -> Translation/Trigger

== system Model_TranslationEngine64/ModelPreAmp/DecRate/Medusa5H1/MedusaHoligram/Medusa5H1 Part 3/On/Expand Tail Components/Tail Component EQ/InnerLink ==
  PoolIirTunableWithReset : Subsystem  mask(Bose Pool IIR Tunable){FeatureName=tailCompEQ, Config=Config}
      mask prompts: FeatureName "Filter name/purpose"; Config "PoolIirTunableWithResetConfig"
      mask help:
      | Pool IIR Tunable is a configurable multi-channel IIR filter that supports one or more channels. This block offers flexibility of tuning the number of stages and coefficients. Different filter coefficients and number of stages (biquads) can be used for each channel filter. The Pool IIR Tunable block supports different implementations, which could be configured at build-time:
      |
      | (i)   Generic: IIR filter code not optimized for any processor
      | (ii)  SharcCore: IIR filters executing on core (uses pooliir.asm CRL)
      | (iii) SharcGulAccel: IIR filters executing on IIR hardware accelerator, offloading MIPS usage from core
      | (iv) SharcGxpAccel: IIR filters take advantage of additional accelerators available on GXP processor
      | (v)  Hexagon: TBD
      |
      | NOTE: When using Pool IIR for Sharc-plus based processors, the codeWorkMemory buffer and input buffer should always be mapped to L1 memory to optimize MIPS utilization and avoid audio artifacts.
      |
      | For more information, please see 'Help'.
      mask init:
      | blkh=gcbh;
      | Config=BTConfig.Assert(blkh,Config);
      | 
      | BTConfig.InitSetFeatureIfPresent(blkh,'FeatureName');
      | Config.Validate();
      | Config.DoMaskInit(blkh);
      mask Help:
      | <b>Input signals: </b>
      | AudioIn: input channels [frame size x number of channels]
      | ResetTrigger: trigger to reset internal state buffer (usually preferred as a post RMDL step)
      | 
      | <b>Output signals: </b>
      | AudioOut: output channels [frame size x number of channels]
      | 
      | <b>Mask parameters: </b>
      | PoolIirTunableWithResetConfig
      | Filter name/purpose
      mask TypeOptions FeatureName: FeaturePath/FeatureName
      mask Callback Config: BTConfig.CallbackHideIfPresent(gcbh,{'FeatureName'});
      mask Display: DrawPoolIirIcon;

== system Model_TranslationEngine64/ModelPreAmp/DecRate/Medusa5H1/MedusaHoligram/Medusa5H1 Part 3/On/Full-rate Mixer/Full-Rate Mixer with CAE & Fade Ramper/Fade Tuning ==
  Backward Downmix Max : Subsystem  Description=This is the fraction of downmixing that occurs when 100% fade (back) is reached.
  Backward Downmix Threshold : Subsystem  Description=This is the fraction of fade (back) at which downmixing of premix coefficients starts.
  Downmix Weights CS : Subsystem  Description=These are the mixing weights at fader extreme when downmix_max is set to 1.
  Downmix Weights Left : Subsystem  Description=These are the mixing weights at fader extreme when downmix_max is set to 1.
  Downmix Weights Right : Subsystem  Description=These are the mixing weights at fader extreme when downmix_max is set to 1.
  Forward Downmix Threshold : Subsystem  Description=This is the fraction of fade (front) at which downmixing of premix coefficients starts.
  Foward Downmix Max : Subsystem  Description=This is the fraction of downmixing that occurs when 100% fade (front) is reached.

== system Model_TranslationEngine64/ModelPreAmp/DecRate/Medusa5H1/MedusaHoligram/Medusa5H1 Part 3/On/Full-rate Mixer/Full-Rate Mixer with CAE & Fade Ramper/SLC Tuning ==
  Detent Level CS : Subsystem  Description="This is the premix (scalar mixing) matrix for the detent (default) level of \"surroundiness\"."
  Detent Level Left : Subsystem  Description="This is the premix (scalar mixing) matrix for the detent (default) level of \"surroundiness\"."
  Detent Level Right : Subsystem  Description="This is the premix (scalar mixing) matrix for the detent (default) level of \"surroundiness\"."
  Interpolation Method : Subsystem  Description=|
      | This controls the method used to interpolate premix coefficient matrix as the surround knob is adjusted.
      | - 0 for linear interpolation (default)
      | - 1 for db-linear interpolation
  Max Level CS : Subsystem  Description="This is the premix (scalar mixing) matrix for the maximum level of \"surroundiness\"."
  Max Level Left : Subsystem  Description="This is the premix (scalar mixing) matrix for the maximum level of \"surroundiness\"."
  Max Level Right : Subsystem  Description="This is the premix (scalar mixing) matrix for the maximum level of \"surroundiness\"."
  Min Level CS : Subsystem  Description="This is the premix (scalar mixing) matrix for the minimum level of \"surroundiness\" i.e. steroe case."
  Min Level Left : Subsystem  Description="This is the premix (scalar mixing) matrix for the minimum level of \"surroundiness\" i.e. steroe case."
  Min Level Right : Subsystem  Description="This is the premix (scalar mixing) matrix for the minimum level of \"surroundiness\" i.e. steroe case."

== system Model_TranslationEngine64/ModelPreAmp/DecRate/Medusa5H1/MedusaHoligram/Medusa5H1 Part 3/On/Premix/Premix with Mono-Surround & CAE with Fade Ramper/CS Processing ==
  FeaturePath : FeaturePath/FeaturePath  FeatureName=MonoSurround  IsGroup=off  GroupNumber=-1  IsModule=off  TriggerInit=[310 264 425 371]
      settings: SourceProductName=Bose Talaria
  MS Tune : Subsystem

== system Model_TranslationEngine64/ModelPreAmp/DecRate/Medusa5H1/MedusaHoligram/Medusa5H1 Part 3/On/Premix/Premix with Mono-Surround & CAE with Fade Ramper/Fade Tuning ==
  Backward Downmix Max : Subsystem  Description=This is the fraction of downmixing that occurs when 100% fade (back) is reached.
  Backward Downmix Threshold : Subsystem  Description=This is the fraction of fade (back) at which downmixing of premix coefficients starts.
  Downmix Weights CS : Subsystem  Description=These are the mixing weights at fader extreme when downmix_max is set to 1.
  Downmix Weights Left : Subsystem  Description=These are the mixing weights at fader extreme when downmix_max is set to 1.
  Downmix Weights Right : Subsystem  Description=These are the mixing weights at fader extreme when downmix_max is set to 1.
  Forward Downmix Threshold : Subsystem  Description=This is the fraction of fade (front) at which downmixing of premix coefficients starts.
  Foward Downmix Max : Subsystem  Description=This is the fraction of downmixing that occurs when 100% fade (front) is reached.

== system Model_TranslationEngine64/ModelPreAmp/DecRate/Medusa5H1/MedusaHoligram/Medusa5H1 Part 3/On/Premix/Premix with Mono-Surround & CAE with Fade Ramper/SLC Tuning ==
  Detent Level CS : Subsystem  Description="This is the premix (scalar mixing) matrix for the detent (default) level of \"surroundiness\"."
  Detent Level Left : Subsystem  Description="This is the premix (scalar mixing) matrix for the detent (default) level of \"surroundiness\"."
  Detent Level Right : Subsystem  Description="This is the premix (scalar mixing) matrix for the detent (default) level of \"surroundiness\"."
  Interpolation Method : Subsystem  Description=|
      | This controls the method used to interpolate premix coefficient matrix as the surround knob is adjusted.
      | - 0 for linear interpolation (default)
      | - 1 for db-linear interpolation
  Max Level CS : Subsystem  Description="This is the premix (scalar mixing) matrix for the maximum level of \"surroundiness\"."
  Max Level Left : Subsystem  Description="This is the premix (scalar mixing) matrix for the maximum level of \"surroundiness\"."
  Max Level Right : Subsystem  Description="This is the premix (scalar mixing) matrix for the maximum level of \"surroundiness\"."
  Min Level CS : Subsystem  Description="This is the premix (scalar mixing) matrix for the minimum level of \"surroundiness\" i.e. steroe case."
  Min Level Left : Subsystem  Description="This is the premix (scalar mixing) matrix for the minimum level of \"surroundiness\" i.e. steroe case."
  Min Level Right : Subsystem  Description="This is the premix (scalar mixing) matrix for the minimum level of \"surroundiness\" i.e. steroe case."

== system Model_TranslationEngine64/ModelPreAmp/DecRate/Medusa5H1/MedusaHoligram/Medusa5H1 Part 3/On/VLS Gains Computation/VLS Gains Drv/Fade Tuning ==
  Backward Downmix Max : Subsystem  Description=This is the fraction of downmixing that occurs when 100% fade (back) is reached.
  Backward Downmix Threshold : Subsystem  Description=This is the fraction of fade (back) at which downmixing of premix coefficients starts.
  Downmix Weights : Subsystem  Description=These are the mixing weights at fader extreme when downmix_max is set to 1.
  Forward Downmix Threshold : Subsystem  Description=This is the fraction of fade (front) at which downmixing of premix coefficients starts.
  Foward Downmix Max : Subsystem  Description=This is the fraction of downmixing that occurs when 100% fade (front) is reached.

== system Model_TranslationEngine64/ModelPreAmp/DecRate/Medusa5H1/MedusaHoligram/Medusa5H1 Part 3/On/VLS Gains Computation/VLS Gains Drv/SLC Tuning ==
  Detent Level : Subsystem  Description="This is the premix (scalar mixing) matrix for the detent (default) level of \"surroundiness\"."
  Interpolation Method : Subsystem  Description=|
      | This controls the method used to interpolate premix coefficient matrix as the surround knob is adjusted.
      | - 0 for linear interpolation (default)
      | - 1 for db-linear interpolation
  Max Level : Subsystem  Description="This is the premix (scalar mixing) matrix for the maximum level of \"surroundiness\"."
  Min Level : Subsystem  Description="This is the premix (scalar mixing) matrix for the minimum level of \"surroundiness\" i.e. steroe case."

== system Model_TranslationEngine64/ModelPreAmp/DecRate/Medusa5H1/MedusaHoligram/Medusa5H1 Part 3/On/VLS Gains Computation/VLS Gains Pax/Fade Tuning ==
  Backward Downmix Max : Subsystem  Description=This is the fraction of downmixing that occurs when 100% fade (back) is reached.
  Backward Downmix Threshold : Subsystem  Description=This is the fraction of fade (back) at which downmixing of premix coefficients starts.
  Downmix Weights : Subsystem  Description=These are the mixing weights at fader extreme when downmix_max is set to 1.
  Forward Downmix Threshold : Subsystem  Description=This is the fraction of fade (front) at which downmixing of premix coefficients starts.
  Foward Downmix Max : Subsystem  Description=This is the fraction of downmixing that occurs when 100% fade (front) is reached.

== system Model_TranslationEngine64/ModelPreAmp/DecRate/Medusa5H1/MedusaHoligram/Medusa5H1 Part 3/On/VLS Gains Computation/VLS Gains Pax/SLC Tuning ==
  Detent Level : Subsystem  Description="This is the premix (scalar mixing) matrix for the detent (default) level of \"surroundiness\"."
  Interpolation Method : Subsystem  Description=|
      | This controls the method used to interpolate premix coefficient matrix as the surround knob is adjusted.
      | - 0 for linear interpolation (default)
      | - 1 for db-linear interpolation
  Max Level : Subsystem  Description="This is the premix (scalar mixing) matrix for the maximum level of \"surroundiness\"."
  Min Level : Subsystem  Description="This is the premix (scalar mixing) matrix for the minimum level of \"surroundiness\" i.e. steroe case."
